simulink model "AntriebeW_V3"  (Simulink 7.6)
settings: Solver=ode45  StartTime=0.0  StopTime=SimulTime  RelTol=1e-3
values from neighbouring files (symbols this model uses):
  f3 = 0.325    [ParamtersAntriebeW.m]
  geometrie = l    (= 0.314159265359)    [ParamtersAntriebeW.m]
  hsp = 200    [ParamtersAntriebeW.m]
  Kraft = 100    [ParamtersAntriebeW.m]
  MaxDrehmoment = 38    [ParamtersAntriebeW.m]
  MaxDrehzahl = 3000    [ParamtersAntriebeW.m]
  PR = 25    [ParamtersAntriebeW.m]
  Pr = 0.7    [ParamtersAntriebeW.m]
  r = 0.2    [ParamtersAntriebeW.m]
  sb = 5.67*(10^-8)    (= 5.67e-08)    [ParamtersAntriebeW.m]
  T_Umgebung = 295    [ParamtersAntriebeW.m]
  Vorschub = 1    [ParamtersAntriebeW.m]
undefined symbols (not defined in the file or in its folder): A, Antriebe, KinematischeViskositaet, m, Temperatur, Waermeleitfaehigkeit
settings Model: Creator=Coni  LastModifiedBy=conid

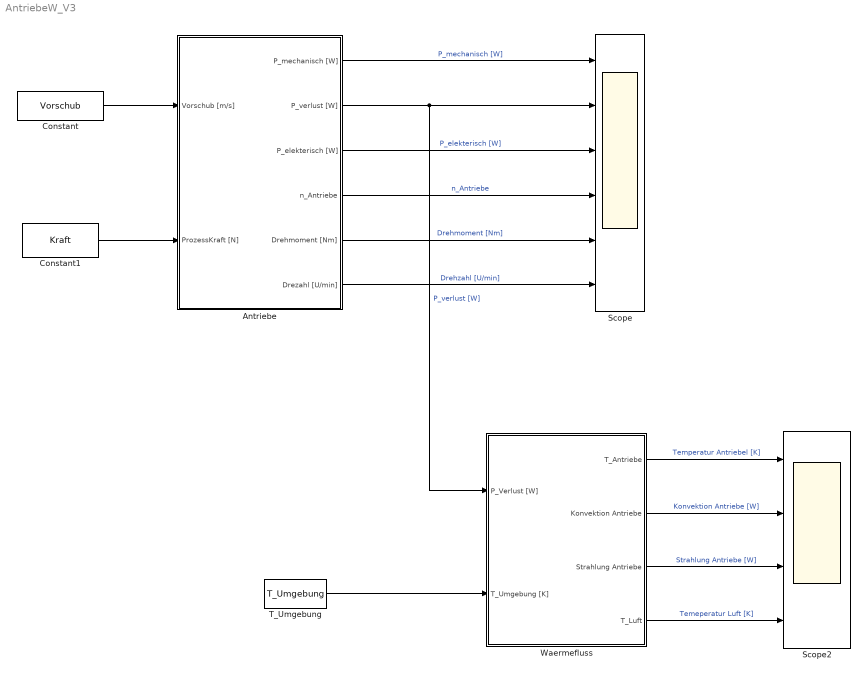
== system AntriebeW_V3 ==
  Antriebe : Subsystem  TreatAsAtomicUnit=on
  Constant : Constant  Value=Vorschub
  Constant1 : Constant  Value=Kraft
  Scope : Scope  NumInputPorts=6
      settings: TimeRange=4  YMin=39520~2.3624e+012~2.3624e+012~1.7595e-008~-5~-5  YMax=43680~2.3643e+012~2.3643e+012~1.7609e-008~5~5  SaveName=Scp_Antriebe
  Scope2 : Scope  NumInputPorts=4
      settings: YMin=306~9.8~13.25~299  YMax=314~10.25~14.75~306  SaveName=Scp_Waermefluss
  T_Umgebung : Constant  Value=T_Umgebung
  Waermefluss : Subsystem  TreatAsAtomicUnit=on
  wires:
  Constant/1 -> Antriebe/1(Vorschub [m/s])
  Constant1/1 -> Antriebe/2(ProzessKraft [N])
  Antriebe/1(P_mechanisch [W]) -> Scope/1  "P_mechanisch [W]"
  Antriebe/4(n_Antriebe) -> Scope/4  "n_Antriebe"
  Antriebe/2(P_verlust [W]) -> Scope/2, Waermefluss/1(P_Verlust [W])  "P_verlust [W]"
  Antriebe/3(P_elekterisch [W]) -> Scope/3  "P_elekterisch [W]"
  Antriebe/5(Drehmoment [Nm]) -> Scope/5  "Drehmoment [Nm]"
  Antriebe/6(Drezahl [U/min]) -> Scope/6  "Drehzahl [U/min]"
  T_Umgebung/1 -> Waermefluss/2(T_Umgebung [K])
  Waermefluss/1(T_Antriebe) -> Scope2/1  "Temperatur Antriebel [K]"
  Waermefluss/2("Konvektion Antriebe ") -> Scope2/2  "Konvektion Antriebe [W]"
  Waermefluss/3(Strahlung Antriebe) -> Scope2/3  "Strahlung Antriebe [W]"
  Waermefluss/4(T_Luft) -> Scope2/4  "Temeperatur Luft [K]"

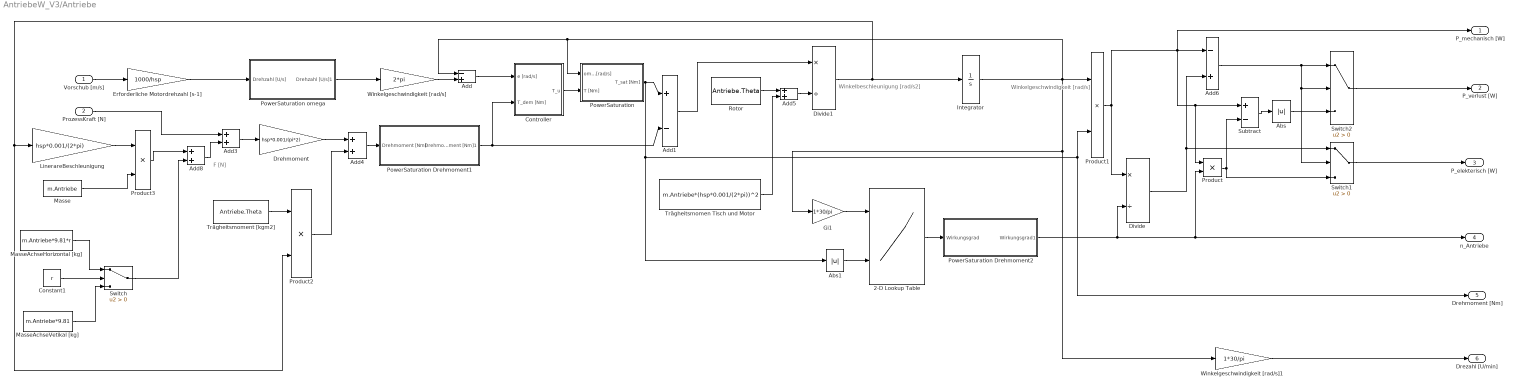
== system AntriebeW_V3/Antriebe ==
  note: Winkelgeschwindigkeit [rad/s]
  note: F [N]
  note: Winkelbeschleunigung [rad/s2]
  Vorschub [m/s] : Inport
  ProzessKraft [N] : Inport  Port=2
  2-D Lookup Table : Lookup_n-D  BreakpointsForDimension1=Antriebe.Tabelomega  BreakpointsForDimension2=Antriebe.TabelM  BreakpointsForDimension1Min=[0]  BreakpointsForDimension2Min=[0]  BreakpointsForDimension1Max=[3000]  BreakpointsForDimension2Max=[9.5]  Table=Antriebe.Tabeleta  TableMin=[0]  TableMax=[1]  InterpMethod=Cubic spline  ExtrapMethod=None - Clip  OutMin=[0]  OutMax=[1]  RndMeth=Simplest  InputSameDT=on
  Abs : Abs
  Abs1 : Abs
  Add : Sum  Inputs=-+
  Add1 : Sum  Inputs=+-
  Add{3..5,8} (4 alike) : Sum
  Add6 : Sum  Inputs=-+
  Constant1 : Constant  Value=r
  Controller : Subsystem  TreatAsAtomicUnit=on
  Divide : Product  Inputs=*/
  Divide1 : Product  Inputs=*/
  Drehmoment : Gain  Gain=hsp*0.001/(pi*2)
  Erforderliche Motordrehzahl [s-1] : Gain  Gain=1000/hsp
  Gi1 : Gain  Gain=1*30/pi
  Integrator : Integrator
  LinerareBeschleunigung : Gain  Gain=hsp*0.001/(2*pi)
  Masse : Constant  Value=m.Antriebe
  MasseAchseHorizontal [kg] : Constant  Value=m.Antriebe*9.81*r
  MasseAchseVetikal [kg] : Constant  Value=m.Antriebe*9.81
  PowerSaturation : Subsystem  TreatAsAtomicUnit=on
  PowerSaturation Drehmoment1 : Subsystem  TreatAsAtomicUnit=on
  PowerSaturation Drehmoment2 : Subsystem  TreatAsAtomicUnit=on
  PowerSaturation omega : Subsystem  TreatAsAtomicUnit=on
  Product{,1..3} (4 alike) : Product  RndMeth=Zero
  Rotor : Constant  Value=Antriebe.Theta
  Subtract : Sum  Inputs=+-
  Switch : Switch  Criteria=u2 > Threshold
  Switch1 : Switch  Criteria=u2 > Threshold
  Switch2 : Switch  Criteria=u2 > Threshold
  Trägheitsmomen Tisch und Motor : Constant  Value=m.Antriebe*(hsp*0.001/(2*pi))^2
  Trägheitsmoment [kgm2] : Constant  Value=Antriebe.Theta
  Winkelgeschwindigkeit [rad/s] : Gain  Gain=2*pi
  Winkelgeschwindigkeit [rad/s]1 : Gain  Gain=1*30/pi
  P_mechanisch [W] : Outport
  P_verlust [W] : Outport  Port=2
  P_elekterisch [W] : Outport  Port=3
  n_Antriebe : Outport  Port=4
  Drehmoment [Nm] : Outport  Port=5
  Drezahl [U/min] : Outport  Port=6
  wires:
  Add/1 -> Controller/1(e [rad/s])
  Controller/1(T_u) -> PowerSaturation/2(T [Nm])
  PowerSaturation/1(T_sat [Nm]) -> Add1/1, Abs1/1, Product1/2, Drehmoment [Nm]/1
  Divide1/1 -> Integrator/1, Product2/2, LinerareBeschleunigung/1
  Integrator/1 -> Add/1, PowerSaturation/1(omega [rad/s]), Product1/1, Gi1/1, Winkelgeschwindigkeit [rad/s]1/1
  Product1/1 -> Divide/1, Add6/1, P_mechanisch [W]/1, Subtract/1, Product/1
  Gi1/1 -> 2-D Lookup Table/1
  Winkelgeschwindigkeit [rad/s]/1 -> Add/2
  Add1/1 -> Divide1/1
  Add3/1 -> Drehmoment/1
  Drehmoment/1 -> Add4/1
  ProzessKraft [N]/1 -> Add3/1
  Add5/1 -> Divide1/2
  Rotor/1 -> Add5/1
  Trägheitsmoment [kgm2]/1 -> Product2/1
  Product2/1 -> Add4/2
  MasseAchseHorizontal [kg]/1 -> Switch/1
  MasseAchseVetikal [kg]/1 -> Switch/3
  Constant1/1 -> Switch/2
  Vorschub [m/s]/1 -> Erforderliche Motordrehzahl [s-1]/1
  Trägheitsmomen Tisch und Motor/1 -> Add5/2
  Add8/1 -> Add3/2
  Switch/1 -> Add8/2
  Masse/1 -> Product3/2
  Product3/1 -> Add8/1
  LinerareBeschleunigung/1 -> Product3/1
  Add6/1 -> Switch2/1, Switch2/2, Switch1/2
  Product/1 -> Subtract/2, Switch1/3
  Subtract/1 -> Abs/1
  Abs/1 -> Switch2/3
  Divide/1 -> Add6/2, Switch1/1
  Switch1/1 -> P_elekterisch [W]/1
  Switch2/1 -> P_verlust [W]/1
  Add4/1 -> PowerSaturation Drehmoment1/1(Drehmoment [Nm])
  PowerSaturation Drehmoment1/1(Drehmoment [Nm]1) -> Controller/2(T_dem [Nm]), Add1/2
  Abs1/1 -> 2-D Lookup Table/2
  Winkelgeschwindigkeit [rad/s]1/1 -> Drezahl [U/min]/1
  Erforderliche Motordrehzahl [s-1]/1 -> PowerSaturation omega/1(Drehzahl [U/s])
  PowerSaturation omega/1(Drehzahl [U/s]1) -> Winkelgeschwindigkeit [rad/s]/1
  2-D Lookup Table/1 -> PowerSaturation Drehmoment2/1(Wirkungsgrad)
  PowerSaturation Drehmoment2/1(Wirkungsgrad1) -> Divide/2, n_Antriebe/1, Product/2

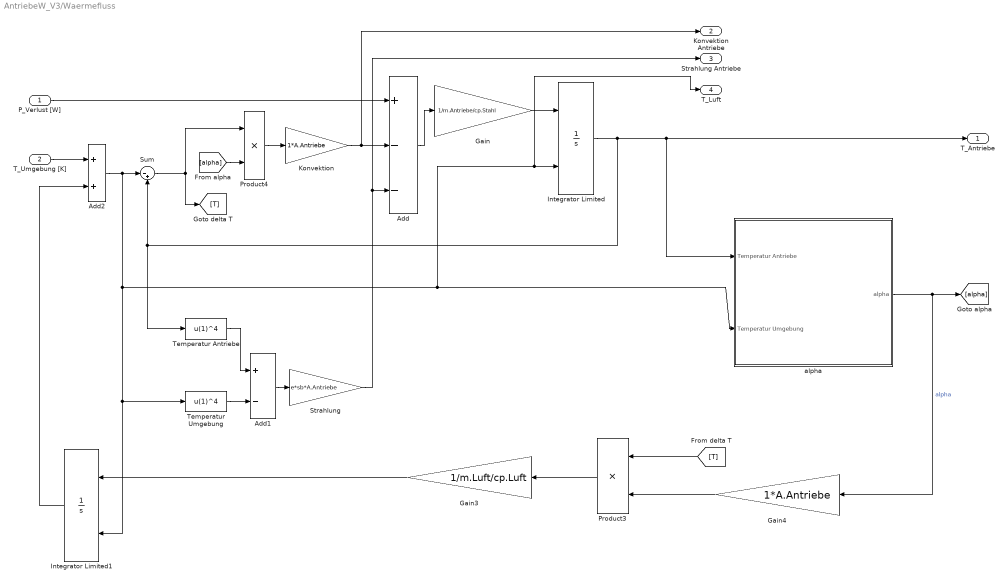
== system AntriebeW_V3/Waermefluss ==
  P_Verlust [W] : Inport
  T_Umgebung [K] : Inport  Port=2
  Add : Sum  Inputs=+--
  Add1 : Sum  Inputs=+-
  Add2 : Sum
  Gain : Gain  Gain=1/m.Antriebe/cp.Stahl
  Gain3 : Gain  Gain=1/m.Luft/cp.Luft
  Gain4 : Gain  Gain=1*A.Antriebe
  Integrator Limited : Integrator  InitialConditionSource=external  LimitOutput=on  ZeroCross=off
  Integrator Limited1 : Integrator  InitialConditionSource=external  LimitOutput=on  ZeroCross=off
  Konvektion : Gain  Gain=1*A.Antriebe
  Product3 : Product  RndMeth=Zero
  Product4 : Product  RndMeth=Zero
  Strahlung : Gain  Gain=e*sb*A.Antriebe
  Sum : Sum  Inputs=|-+
  Temperatur Antriebe : Fcn  Expr=u(1)^4
  Temperatur Umgebung : Fcn  Expr=u(1)^4
  alpha : Subsystem
  T_Antriebe : Outport
  "Konvektion Antriebe " : Outport  Port=2
  Strahlung Antriebe : Outport  Port=3
  T_Luft : Outport  Port=4
  wires:
  P_Verlust [W]/1 -> Add/1
  Sum/1 -> Product4/1, [T]
  Gain/1 -> Integrator Limited/1
  Konvektion/1 -> Add/2, "Konvektion Antriebe "/1
  Integrator Limited/1 -> T_Antriebe/1, alpha/1(Temperatur Antriebe), Sum/2, Temperatur Antriebe/1
  Add/1 -> Gain/1
  Strahlung/1 -> Strahlung Antriebe/1, Add/3
  Temperatur Antriebe/1 -> Add1/1
  Add1/1 -> Strahlung/1
  Add2/1 -> Sum/1, Integrator Limited/2, T_Luft/1, alpha/2(Temperatur Umgebung), Integrator Limited1/2, Temperatur Umgebung/1
  T_Umgebung [K]/1 -> Add2/1
  Product4/1 -> Konvektion/1
  [alpha] -> Product4/2
  Integrator Limited1/1 -> Add2/2
  Gain3/1 -> Integrator Limited1/1
  Temperatur Umgebung/1 -> Add1/2
  alpha/1(alpha) -> [alpha], Gain4/1  "alpha"
  Gain4/1 -> Product3/2
  Product3/1 -> Gain3/1
  [T] -> Product3/1

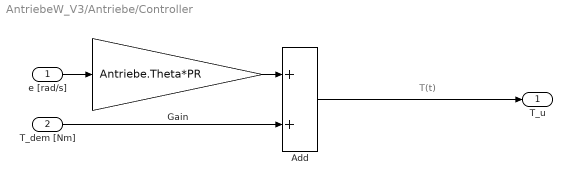
== system AntriebeW_V3/Antriebe/Controller ==
  note: T(t)
  e [rad/s] : Inport
  T_dem [Nm] : Inport  Port=2
  Add : Sum
  Gain : Gain  Gain=Antriebe.Theta*PR
  T_u : Outport
  wires:
  Add/1 -> T_u/1
  T_dem [Nm]/1 -> Add/2
  Gain/1 -> Add/1
  e [rad/s]/1 -> Gain/1

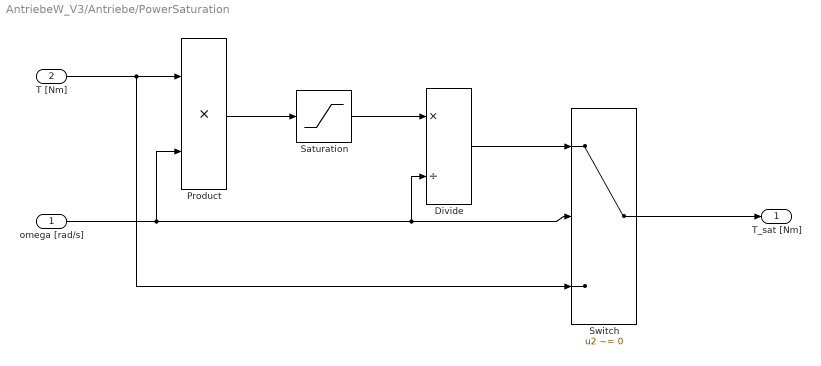
== system AntriebeW_V3/Antriebe/PowerSaturation ==
  omega [rad/s] : Inport
  T [Nm] : Inport  Port=2
  Divide : Product  Inputs=*/
  Product : Product  RndMeth=Zero
  Saturation : Saturate  UpperLimit=Antriebe.Pmax  LowerLimit=-Antriebe.Pmax  ZeroCross=off
  Switch : Switch  Criteria=u2 ~= 0
  T_sat [Nm] : Outport
  wires:
  Product/1 -> Saturation/1
  Saturation/1 -> Divide/1
  Divide/1 -> Switch/1
  Switch/1 -> T_sat [Nm]/1
  T [Nm]/1 -> Product/1, Switch/3
  omega [rad/s]/1 -> Switch/2, Divide/2, Product/2

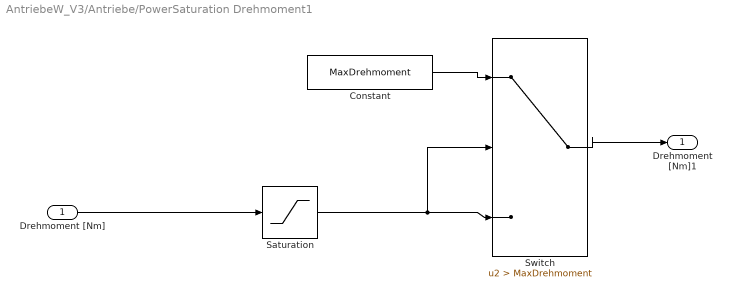
== system AntriebeW_V3/Antriebe/PowerSaturation Drehmoment1 ==
  Drehmoment [Nm] : Inport
  Constant : Constant  Value=MaxDrehmoment
  Saturation : Saturate  UpperLimit=9.5  LowerLimit=-9.5  ZeroCross=off
  Switch : Switch  Criteria=u2 > Threshold  Threshold=MaxDrehmoment
  Drehmoment [Nm]1 : Outport
  wires:
  Saturation/1 -> Switch/3, Switch/2
  Constant/1 -> Switch/1
  Drehmoment [Nm]/1 -> Saturation/1
  Switch/1 -> Drehmoment [Nm]1/1

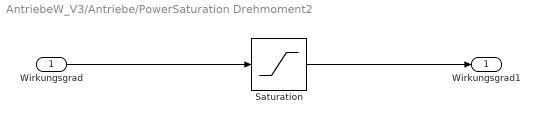
== system AntriebeW_V3/Antriebe/PowerSaturation Drehmoment2 ==
  Wirkungsgrad : Inport
  Saturation : Saturate  UpperLimit=0.95  LowerLimit=0.1  ZeroCross=off
  Wirkungsgrad1 : Outport
  wires:
  Wirkungsgrad/1 -> Saturation/1
  Saturation/1 -> Wirkungsgrad1/1

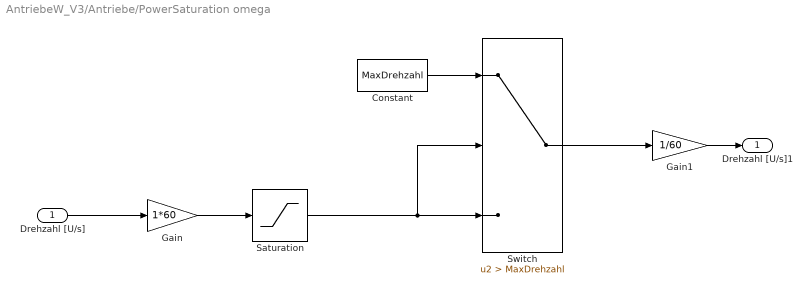
== system AntriebeW_V3/Antriebe/PowerSaturation omega ==
  Drehzahl [U/s] : Inport
  Constant : Constant  Value=MaxDrehzahl
  Gain : Gain  Gain=1*60
  Gain1 : Gain  Gain=1/60
  Saturation : Saturate  UpperLimit=MaxDrehzahl  LowerLimit=0  ZeroCross=off
  Switch : Switch  Criteria=u2 > Threshold  Threshold=MaxDrehzahl
  Drehzahl [U/s]1 : Outport
  wires:
  Saturation/1 -> Switch/3, Switch/2
  Constant/1 -> Switch/1
  Drehzahl [U/s]/1 -> Gain/1
  Gain/1 -> Saturation/1
  Gain1/1 -> Drehzahl [U/s]1/1
  Switch/1 -> Gain1/1

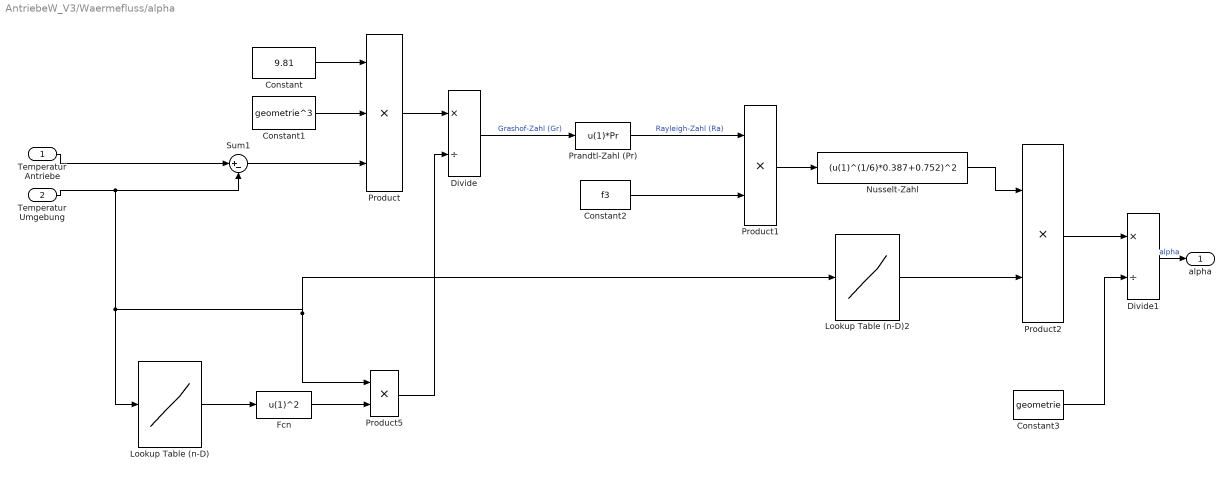
== system AntriebeW_V3/Waermefluss/alpha ==
  Temperatur Antriebe : Inport
  Temperatur Umgebung : Inport  Port=2
  Constant : Constant  Value=9.81
  Constant1 : Constant  Value=geometrie^3
  Constant2 : Constant  Value=f3
  Constant3 : Constant  Value=geometrie
  Divide : Product  Inputs=*/
  Divide1 : Product  Inputs=*/
  Fcn : Fcn  Expr=u(1)^2
  Lookup Table (n-D) : Lookup_n-D  NumberOfTableDimensions=1  BreakpointsForDimension1=Temperatur.Tabel  Table=KinematischeViskositaet.Tabel  InterpMethod=Cubic spline  ExtrapMethod=None - Clip  InputSameDT=on
  Lookup Table (n-D)2 : Lookup_n-D  NumberOfTableDimensions=1  BreakpointsForDimension1=Temperatur.Tabel  Table=Waermeleitfaehigkeit.Tabel  InterpMethod=Cubic spline  ExtrapMethod=None - Clip  InputSameDT=on
  Nusselt-Zahl : Fcn  Expr=(u(1)^(1/6)*0.387+0.752)^2
  Prandtl-Zahl (Pr) : Fcn  Expr=u(1)*Pr
  Product : Product  Inputs=3  RndMeth=Zero
  Product1 : Product  RndMeth=Zero
  Product2 : Product  RndMeth=Zero
  Product5 : Product  RndMeth=Zero
  Sum1 : Sum  Inputs=|+-
  alpha : Outport
  wires:
  Constant/1 -> Product/1
  Constant1/1 -> Product/2
  Sum1/1 -> Product/3
  Product/1 -> Divide/1
  Divide/1 -> Prandtl-Zahl (Pr)/1  "Grashof-Zahl (Gr)"
  Prandtl-Zahl (Pr)/1 -> Product1/1  "Rayleigh-Zahl (Ra)"
  Constant2/1 -> Product1/2
  Lookup Table (n-D)2/1 -> Product2/2
  Product2/1 -> Divide1/1
  Divide1/1 -> alpha/1  "alpha"
  Product5/1 -> Divide/2
  Lookup Table (n-D)/1 -> Fcn/1
  Fcn/1 -> Product5/2
  Product1/1 -> Nusselt-Zahl/1
  Nusselt-Zahl/1 -> Product2/1
  Constant3/1 -> Divide1/2
  Temperatur Antriebe/1 -> Sum1/1
  Temperatur Umgebung/1 -> Sum1/2, Lookup Table (n-D)/1, Product5/1, Lookup Table (n-D)2/1
